simulink model "UAV"  (R2024a)
settings: Solver=FixedStepAuto  StartTime=0  StopTime=inf  MaxStep=0.01  RelTol=1e-4
values from neighbouring files (symbols this model uses):
  actuatorCentres = 0.0    [data.sldd]
  datcom1 : value not decoded    [data.sldd]
  deflectionLimits = -10.0    [data.sldd]
  loggingSampleTime = 1.0    [data.sldd]
  sensorSampleTime = 0.02    [data.sldd]
  vehicle = 1.23    [data.sldd]
undefined symbols (not defined in the file or in its folder): aeroCoeff, aMode, DiscIntNeverNeededParam, Discrete, Earth, HDBK, MIL, Newton, pa28, Raphson, Time, WGS84
libraries: slpidlib x20, simulink_extras x15, simulink x13, arduinolib x8, aerolibasang x5, aerolibactuator x4, aerolibutil x4, aerolibtransform2 x4, sharedtransform x3, ctrlSharedLib x3, aerolibadyn x3, dspstat3 x2
(part 5 of 5)

== system UAV/Arduino/Sensors/Real Sensors/LLA to Flat Earth1/LatLong wrap LL0/Latitude Wrap 90 ==
  Lat : Inport
  Abs1 : Abs  SaturateOnIntegerOverflow=off
  Bias : Bias  Bias=-90  SaturateOnIntegerOverflow=off
  Bias1 : Bias  Bias=+90  SaturateOnIntegerOverflow=off
  Compare To Constant : simulink/Logic and Bit Operations/Compare To Constant  relop=>  const=90  OutDataTypeStr=boolean
  Divide1 : Product  Inputs=**
  Gain : Gain  Gain=-1
  Sign1 : Signum
  Switch : Switch  Criteria=u2 ~= 0  SaturateOnIntegerOverflow=off  InputSameDT=off
  Wrap Angle 180 : Subsystem  AncestorBlock=aerolibtransform2sys/Wrap Angle 180
      mask init:
      | aeroicon('aeroblk');
  Lat wrapped : Outport  VectorParamsAs1DForOutWhenUnconnected=off
  Wrap flag : Outport  Port=2  VectorParamsAs1DForOutWhenUnconnected=off
  wires:
  Compare To Constant/1 -> Switch/2, Wrap flag/1
  Wrap Angle 180/1(Angle 180) -> Sign1/1, Switch/3, Abs1/1
  Lat/1 -> Wrap Angle 180/1(Angle)
  Abs1/1 -> Compare To Constant/1, Bias/1
  Bias/1 -> Gain/1
  Gain/1 -> Bias1/1
  Bias1/1 -> Divide1/2
  Sign1/1 -> Divide1/1
  Divide1/1 -> Switch/1
  Switch/1 -> Lat wrapped/1

== system UAV/Arduino/Sensors/Real Sensors/LLA to Flat Earth1/LatLong wrap LL0/Wrap Longitude ==
  Angle : Inport
  Abs : Abs  SaturateOnIntegerOverflow=off
  Bias : Bias  Bias=180  SaturateOnIntegerOverflow=off
  Bias1 : Bias  Bias=-180  SaturateOnIntegerOverflow=off
  Compare To Constant : simulink/Logic and Bit Operations/Compare To Constant  relop=>  const=180  OutDataTypeStr=boolean
  Constant2 : Constant  Value=360  OutDataTypeStr=single
  Math Function1 : Math  Operator=mod  SignedPower=on
  Switch : Switch  Criteria=u2 ~= 0  Threshold=180  SaturateOnIntegerOverflow=off  InputSameDT=off
  Angle 180 : Outport  VectorParamsAs1DForOutWhenUnconnected=off
  wires:
  Compare To Constant/1 -> Switch/2
  Angle/1 -> Bias/1, Switch/3, Abs/1
  Abs/1 -> Compare To Constant/1
  Bias/1 -> Math Function1/1
  Constant2/1 -> Math Function1/2
  Math Function1/1 -> Bias1/1
  Bias1/1 -> Switch/1
  Switch/1 -> Angle 180/1

== system UAV/Arduino/Sensors/Real Sensors/LLA to Flat Earth1/Subsystem1/Subsystem ==
  mu : Inport
  Angle Conversion2 : aerolibtransform2/LLA to Flat Earth/Subsystem/Find Radian//Distance/Angle Conversion2  SystemSampleTime=-1
      settings: SourceProductName=Aerospace Blockset
  Constant : Constant  OutDataTypeStr=single
  Constant1 : Constant  Value=6378137  OutDataTypeStr=single
  Constant2 : Constant  OutDataTypeStr=single
  Constant3 : Constant  OutDataTypeStr=single
  Constant4 : Constant  Value=0.00669437999  OutDataTypeStr=single
  Product1 : Product  Inputs=*/  RndMeth=Zero
  Product3 : Product  Inputs=**/  OutDataTypeStr=single  RndMeth=Zero
  Product4 : Product  RndMeth=Zero
  Subsystem2 : Subsystem
  Sum1 : Sum  Inputs=|+-
  Trigonometric Function : Trigonometry  Operator=cos
  Trigonometric Function1 : Trigonometry  Operator=atan2
  Trigonometric Function2 : Trigonometry  Operator=atan2
  sqrt : Sqrt  AlgorithmType=Newton-Raphson
  dNorth : Outport  VectorParamsAs1DForOutWhenUnconnected=off
  dEast : Outport  Port=2  VectorParamsAs1DForOutWhenUnconnected=off
  wires:
  Angle Conversion2/1 -> Subsystem2/2(mu), Trigonometric Function/1
  Constant/1 -> Sum1/1
  Trigonometric Function2/1 -> dEast/1
  Constant2/1 -> Trigonometric Function1/1
  Constant4/1 -> Sum1/2, Subsystem2/1(eps)
  sqrt/1 -> Product1/2
  Subsystem2/1(denom) -> Product3/3, sqrt/1
  Trigonometric Function/1 -> Product4/2
  Product1/1 -> Product3/1, Product4/1  "Rn"
  Trigonometric Function1/1 -> dNorth/1
  Product3/1 -> Trigonometric Function1/2  "Rm"
  Sum1/1 -> Product3/2
  Product4/1 -> Trigonometric Function2/2
  Constant1/1 -> Product1/1
  Constant3/1 -> Trigonometric Function2/1
  mu/1 -> Angle Conversion2/1

== system UAV/Arduino/Sensors/Real Sensors/Error State Kalman Filter1/Subsystem/Angle Calculation/Protect asincos input ==
  In : Inport
  If : If  IfExpression=u1 > 1  ElseIfExpressions=u1 < -1
  If Action Subsystem : Subsystem  TreatAsAtomicUnit=on
  If Action Subsystem1 : Subsystem  TreatAsAtomicUnit=on
  If Action Subsystem2 : Subsystem  TreatAsAtomicUnit=on
  Merge : Merge  Inputs=3
  Out : Outport  VectorParamsAs1DForOutWhenUnconnected=off
  wires:
  Merge/1 -> Out/1
  If Action Subsystem2/1(OutOrig) -> Merge/3
  If Action Subsystem1/1(OutputNeg1) -> Merge/2
  If Action Subsystem/1(OutputPos1) -> Merge/1
  If/3 -> If Action Subsystem2/Action
  If/2 -> If Action Subsystem1/Action
  In/1 -> If/1, If Action Subsystem2/1(In)
  If/1 -> If Action Subsystem/Action

== system UAV/Arduino/Sensors/Real Sensors/LLA to Flat Earth1/LatLong wrap/Latitude Wrap 90/Wrap Angle 180 ==
  Angle : Inport
  Abs : Abs  SaturateOnIntegerOverflow=off
  Bias : Bias  Bias=180  SaturateOnIntegerOverflow=off
  Bias1 : Bias  Bias=-180  SaturateOnIntegerOverflow=off
  Compare To Constant : simulink/Logic and Bit Operations/Compare To Constant  relop=>  const=180  OutDataTypeStr=boolean
  Constant2 : Constant  Value=360  OutDataTypeStr=single
  Math Function1 : Math  Operator=mod  SignedPower=on
  Switch : Switch  Criteria=u2 ~= 0  Threshold=180  SaturateOnIntegerOverflow=off  InputSameDT=off
  Angle 180 : Outport  VectorParamsAs1DForOutWhenUnconnected=off
  wires:
  Compare To Constant/1 -> Switch/2
  Angle/1 -> Bias/1, Switch/3, Abs/1
  Abs/1 -> Compare To Constant/1
  Bias/1 -> Math Function1/1
  Constant2/1 -> Math Function1/2
  Math Function1/1 -> Bias1/1
  Bias1/1 -> Switch/1
  Switch/1 -> Angle 180/1

== system UAV/Arduino/Sensors/Real Sensors/LLA to Flat Earth1/LatLong wrap LL0/Latitude Wrap 90/Wrap Angle 180 ==
  Angle : Inport
  Abs : Abs  SaturateOnIntegerOverflow=off
  Bias : Bias  Bias=180  SaturateOnIntegerOverflow=off
  Bias1 : Bias  Bias=-180  SaturateOnIntegerOverflow=off
  Compare To Constant : simulink/Logic and Bit Operations/Compare To Constant  relop=>  const=180  OutDataTypeStr=boolean
  Constant : Constant  Value=360  OutDataTypeStr=single
  Math Function1 : Math  Operator=mod  SignedPower=on
  Switch : Switch  Criteria=u2 ~= 0  Threshold=180  SaturateOnIntegerOverflow=off  InputSameDT=off
  Angle 180 : Outport  VectorParamsAs1DForOutWhenUnconnected=off
  wires:
  Compare To Constant/1 -> Switch/2
  Angle/1 -> Bias/1, Switch/3, Abs/1
  Abs/1 -> Compare To Constant/1
  Bias/1 -> Math Function1/1
  Constant/1 -> Math Function1/2
  Math Function1/1 -> Bias1/1
  Bias1/1 -> Switch/1
  Switch/1 -> Angle 180/1

== system UAV/Arduino/Sensors/Real Sensors/LLA to Flat Earth1/Subsystem1/Subsystem/Subsystem2 ==
  eps : Inport
  mu : Inport  Port=2
  Constant : Constant  OutDataTypeStr=single
  Product1 : Product  Inputs=3  OutDataTypeStr=single  RndMeth=Zero
  Sum1 : Sum  Inputs=|+-
  Trigonometric Function1 : Trigonometry
  denom : Outport  VectorParamsAs1DForOutWhenUnconnected=off
  wires:
  Product1/1 -> Sum1/2
  Trigonometric Function1/1 -> Product1/2, Product1/3
  Constant/1 -> Sum1/1
  eps/1 -> Product1/1
  Sum1/1 -> denom/1
  mu/1 -> Trigonometric Function1/1

== system UAV/Arduino/Sensors/Real Sensors/Error State Kalman Filter1/Subsystem/Angle Calculation/Protect asincos input/If Action Subsystem ==
  Action Port : ActionPort  ActionPortLabel=if(u1 > 1)
  Constant : Constant  OutDataTypeStr=single  SampleTime=-1
  OutputPos1 : Outport  InitialOutput=0  VectorParamsAs1DForOutWhenUnconnected=off
  wires:
  Constant/1 -> OutputPos1/1

== system UAV/Arduino/Sensors/Real Sensors/Error State Kalman Filter1/Subsystem/Angle Calculation/Protect asincos input/If Action Subsystem1 ==
  Action Port : ActionPort  ActionPortLabel=elseif(u1 < -1)
  Constant : Constant  OutDataTypeStr=single  SampleTime=-1
  OutputNeg1 : Outport  InitialOutput=0  VectorParamsAs1DForOutWhenUnconnected=off
  wires:
  Constant/1 -> OutputNeg1/1

== system UAV/Arduino/Sensors/Real Sensors/Error State Kalman Filter1/Subsystem/Angle Calculation/Protect asincos input/If Action Subsystem2 ==
  In : Inport
  Action Port : ActionPort  ActionPortLabel=else
  OutOrig : Outport  InitialOutput=0  VectorParamsAs1DForOutWhenUnconnected=off
  wires:
  In/1 -> OutOrig/1

== stateflow chart UAV/Arduino/Flight Control/Real Flight Control/Guidance ==
  settings: executeAtInitialization=1  initializeOutput=1
  state Guidance
    state MAN_OVRDE
    state HDG_Hold
      state HDG
    state HDG_ALT_Hold
      state HDG_ALT
    state ALT_Hold
      state ALT
    (default) -> MAN_OVRDE
    MAN_OVRDE -> HDG_Hold [order 3] : [Demands.FlightMode.HdgHold == 1]
    HDG_ALT_Hold -> MAN_OVRDE [order 3] : [Demands.FlightMode.AltHold == 0 ...
        | && Demands.FlightMode.HdgHold == 0]
    MAN_OVRDE -> HDG_ALT_Hold [order 1] : [Demands.FlightMode.AltHold == 1 ...
        | && Demands.FlightMode.HdgHold == 1]
    HDG_Hold -> MAN_OVRDE [order 3] : [Demands.FlightMode.HdgHold == 0]
    ALT_Hold -> MAN_OVRDE [order 3] : [Demands.FlightMode.AltHold == 0]
    MAN_OVRDE -> ALT_Hold [order 2] : [Demands.FlightMode.AltHold == 1]
    HDG_Hold -> HDG_ALT_Hold [order 1] : [Demands.FlightMode.AltHold == 1 ...
        | && Demands.FlightMode.HdgHold == 1]
    HDG_ALT_Hold -> HDG_Hold [order 2] : [Demands.FlightMode.AltHold == 0 ...
        | && Demands.FlightMode.HdgHold == 1]
    HDG_Hold -> ALT_Hold [order 2] : [Demands.FlightMode.AltHold == 1 ...
        | && Demands.FlightMode.HdgHold == 0]
    ALT_Hold -> HDG_Hold [order 2] : [Demands.FlightMode.AltHold == 0 ...
        | && Demands.FlightMode.HdgHold == 1]
    HDG_ALT_Hold -> ALT_Hold [order 1] : [Demands.FlightMode.AltHold == 1 ...
        | && Demands.FlightMode.HdgHold == 0]
    ALT_Hold -> HDG_ALT_Hold [order 1] : [Demands.FlightMode.AltHold == 1 ...
        | && Demands.FlightMode.HdgHold == 1]
  (default) -> Guidance
  data: sf_internal_action_state_placeholder_data local double size=1 =0; sf_internal_action_state_placeholder_data local double size=1 =0; sf_internal_action_state_placeholder_data local double size=1 =0; Sensors input; Demands input; Commands output size=2

== stateflow chart UAV/Arduino/Flight Control/Model Flight Control/Guidance States ==
  settings: updateMethod=DISCRETE  sampleTime=0.02  executeAtInitialization=1  initializeOutput=1
  state Guidance
    state MAN_OVRDE
    state HDG_Hold
      state HDG
    state HDG_ALT_Hold
      state HDG_ALT
    state ALT_Hold
      state ALT
    (default) -> MAN_OVRDE
    MAN_OVRDE -> HDG_Hold [order 3] : [Demands.FlightMode.HdgHold == 1]
    HDG_ALT_Hold -> MAN_OVRDE [order 3] : [Demands.FlightMode.AltHold == 0 ...
        | && Demands.FlightMode.HdgHold == 0]
    MAN_OVRDE -> HDG_ALT_Hold [order 1] : [Demands.FlightMode.AltHold == 1 ...
        | && Demands.FlightMode.HdgHold == 1]
    HDG_Hold -> MAN_OVRDE [order 3] : [Demands.FlightMode.HdgHold == 0]
    ALT_Hold -> MAN_OVRDE [order 3] : [Demands.FlightMode.AltHold == 0]
    MAN_OVRDE -> ALT_Hold [order 2] : [Demands.FlightMode.AltHold == 1]
    HDG_Hold -> HDG_ALT_Hold [order 1] : [Demands.FlightMode.AltHold == 1 ...
        | && Demands.FlightMode.HdgHold == 1]
    HDG_ALT_Hold -> HDG_Hold [order 2] : [Demands.FlightMode.AltHold == 0 ...
        | && Demands.FlightMode.HdgHold == 1]
    HDG_Hold -> ALT_Hold [order 2] : [Demands.FlightMode.AltHold == 1 ...
        | && Demands.FlightMode.HdgHold == 0]
    ALT_Hold -> HDG_Hold [order 2] : [Demands.FlightMode.AltHold == 0 ...
        | && Demands.FlightMode.HdgHold == 1]
    ALT_Hold -> HDG_ALT_Hold [order 1] : [Demands.FlightMode.AltHold == 1 ...
        | && Demands.FlightMode.HdgHold == 1]
    HDG_ALT_Hold -> ALT_Hold [order 1] : [Demands.FlightMode.AltHold == 1 ...
        | && Demands.FlightMode.HdgHold == 0]
  (default) -> Guidance
  data: sf_internal_action_state_placeholder_data local double size=1 =0; sf_internal_action_state_placeholder_data local double size=1 =0; sf_internal_action_state_placeholder_data local double size=1 =0; Sensors input; Demands input; ControlOverrides input; Cmds output single
